simulink model "airframe"  (R2019b)
settings: Solver=VariableStepAuto  StartTime=0.0  StopTime=10.0  RelTol=1e-3
settings Model: Creator=Alessandro  LastModifiedBy=Alessandro

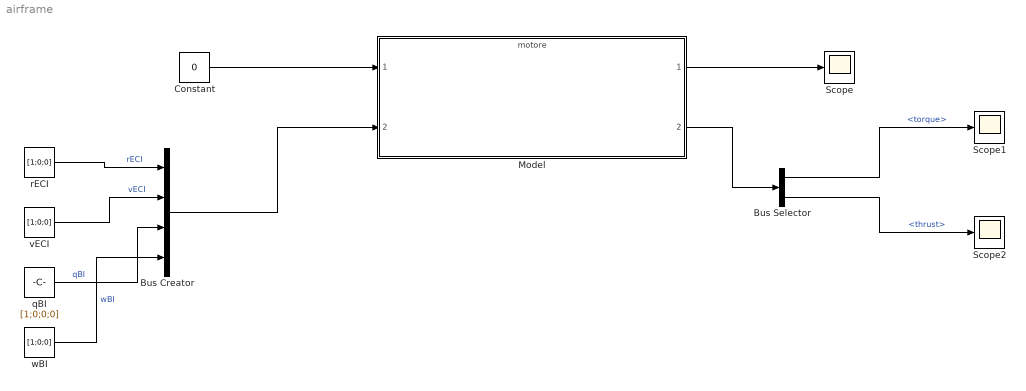
== system airframe ==
  Bus Creator : BusCreator  Inputs=4  OutDataTypeStr=Bus: stato6DoF
      settings: InheritFromInputs=off
  Bus Selector : BusSelector  OutputSignals=torque,thrust
  Constant : Constant  Value=0
  Model : ModelReference  ModelNameDialog=motore  ParameterArgumentNames=C_Q_coeff  ParameterArgumentValues=C_Q_coeff  UsingDefaultArgumentValue=0  SimulationMode=Normal  ModelReferenceVersion=1.5  C_Q_coeff=7  SimulationMode=Normal
  Scope : Scope
  Scope1 : Scope
  Scope2 : Scope
  qBI : Constant  Value=[1;0;0;0]  VectorParams1D=off
  rECI : Constant  Value=[1;0;0]  VectorParams1D=off  OutDataTypeStr=double
  vECI : Constant  Value=[1;0;0]  VectorParams1D=off
  wBI : Constant  Value=[1;0;0]  VectorParams1D=off
  wires:
  Constant/1 -> Model/1
  Bus Creator/1 -> Model/2
  Model/1 -> Scope/1
  Model/2 -> Bus Selector/1
  Bus Selector/1 -> Scope1/1  "<torque>"
  Bus Selector/2 -> Scope2/1  "<thrust>"
  rECI/1 -> Bus Creator/1  "rECI"
  vECI/1 -> Bus Creator/2  "vECI"
  qBI/1 -> Bus Creator/3  "qBI"
  wBI/1 -> Bus Creator/4  "wBI"
